simulink model "MPC4"  (R2020b)
settings: Solver=FixedStepAuto  StartTime=0.0  StopTime=10.0  FixedStep=0.01  RelTol=1e-3  EnableMultiTasking=on
model workspace (MAT data in the model file):
  v0_ego = 1
libraries: autolibshared x1, simulink x1
settings Model: Creator=vicgd  LastModifiedBy=vicgd

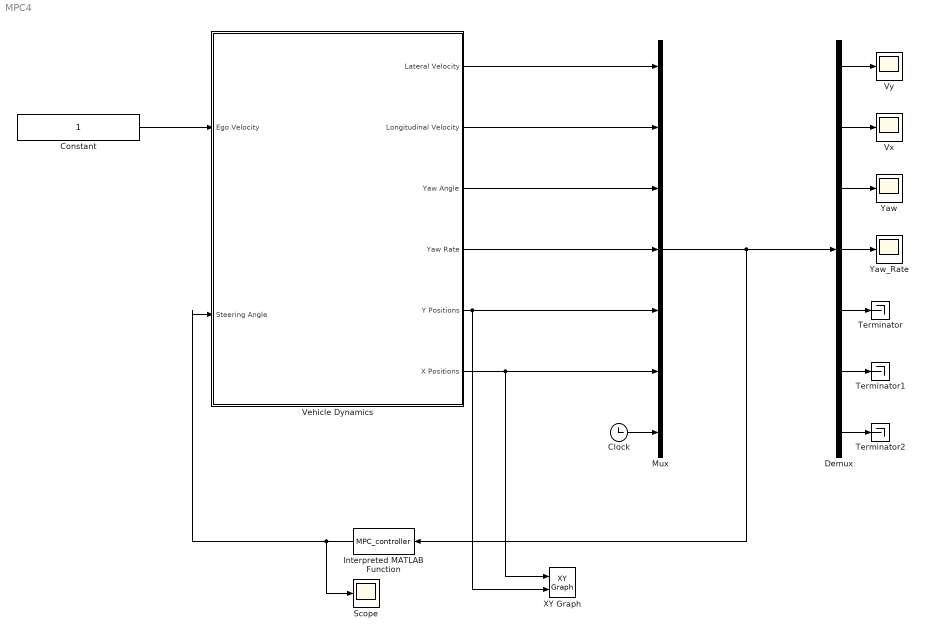
== system MPC4 ==
  Clock : Clock
  Constant : Constant
  Demux : Demux  Outputs=7
  Interpreted MATLAB Function : MATLABFcn  MATLABFcn=MPC_controller  OutputDimensions=1  Output1D=off
  Mux : Mux  Inputs=7
  Scope : Scope
  Terminator : Terminator
  Terminator1 : Terminator
  Terminator2 : Terminator
  Vehicle Dynamics : Subsystem
  Vx : Scope
  Vy : Scope
  XY Graph : simulink/Sinks/XY Graph  xmin=0  xmax=100  ymin=0  ymax=6  st=-1
  Yaw : Scope
  Yaw_Rate : Scope
  wires:
  Mux/1 -> Interpreted MATLAB Function/1, Demux/1
  Clock/1 -> Mux/7
  Vehicle Dynamics/2(Longitudinal Velocity) -> Mux/2
  Vehicle Dynamics/1(Lateral Velocity) -> Mux/1
  Vehicle Dynamics/3(Yaw Angle) -> Mux/3
  Vehicle Dynamics/4(Yaw Rate) -> Mux/4
  Vehicle Dynamics/5(Y Positions) -> XY Graph/2, Mux/5
  Vehicle Dynamics/6(X Positions) -> XY Graph/1, Mux/6
  Demux/1 -> Vy/1
  Demux/2 -> Vx/1
  Demux/3 -> Yaw/1
  Demux/4 -> Yaw_Rate/1
  Interpreted MATLAB Function/1 -> Scope/1, Vehicle Dynamics/2(Steering Angle)
  Constant/1 -> Vehicle Dynamics/1(Ego Velocity)
  Demux/6 -> Terminator1/1
  Demux/7 -> Terminator2/1
  Demux/5 -> Terminator/1

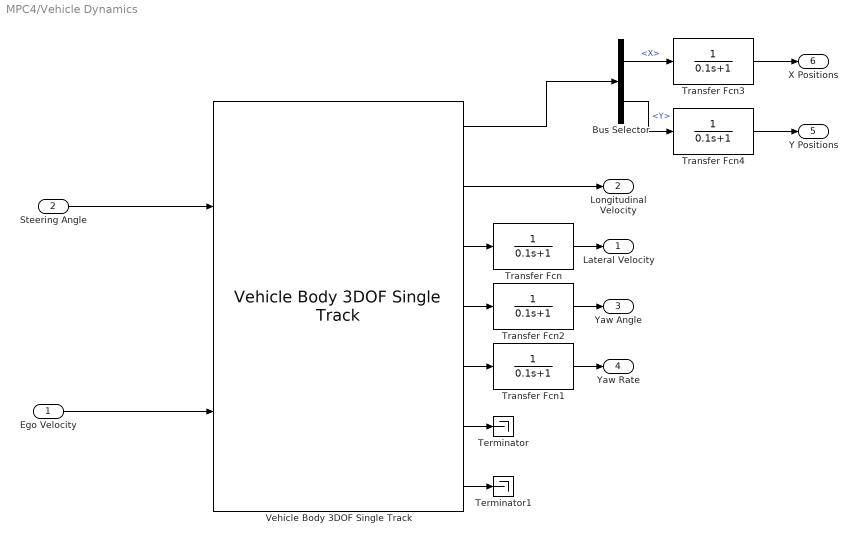
== system MPC4/Vehicle Dynamics ==
  Ego Velocity : Inport
  Steering Angle : Inport  Port=2
  Bus Selector : BusSelector  OutputSignals=InertFrm.Geom.Disp.X,InertFrm.Geom.Disp.Y
  Terminator : Terminator
  Terminator1 : Terminator
  Transfer Fcn{,1..4} (5 alike) : TransferFcn  Denominator=[0.1 1]
  Vehicle Body 3DOF Single Track : autolibshared/Vehicle Body 3DOF Single Track  trackMode=Single (bicycle)  inputMode=External longitudinal velocity  frontSteerMode=on  rearSteerMode=off  windMode=off  muMode=off  extFMode=off  extMMode=off  htchFMode=off  htchMMode=off  extXo=off  extpsio=off  extxdoto=off  extro=off  extYo=off  extTamb=off  extydoto=off  aMode=2  NF=2  NR=2  m=1270  a=1.015  b=1.895  h=0.35  dh=1  hh=0.2  X_o=0  xdot_o=0  CalphaMode=off  sigmaMode=off  d=0  hl=0  w=[1.4,1.4]  Cy_f=1.4e5  Cy_r=8.6e4  sigma_f=.1  sigma_r=.1  alpha_f_brk=[-.1 .1]  Cy_f_data=[-9e3 9e3]  alpha_r_brk=[-.1 .1]  Cy_r_data=[-9e3 9e3]  Y_o=0  ydot_o=0  Izz=1537  psi_o=0  r_o=0  Af=2  Cd=.3  Cl=.1  Cpm=.1  beta_w=[0:0.01:0.3]  Cs=[0:0.03:0.9]  Cym=[0:0.01:0.3]  Pabs=101325  Tair=273  g=9.81  mu=1  xdot_tol=.01  Fznom=5000  Fxtire_sat=7e4  Fytire_sat=7e4  longOff=0  latOff=0  vertOff=0  wrapAng=off
      settings: SourceProductBaseCode=PW,MT,UV,VE,VP
  Lateral Velocity : Outport
  Longitudinal Velocity : Outport  Port=2
  Yaw Angle : Outport  Port=3
  Yaw Rate : Outport  Port=4
  Y Positions : Outport  Port=5
  X Positions : Outport  Port=6
  wires:
  Vehicle Body 3DOF Single Track/3 -> Transfer Fcn/1
  Vehicle Body 3DOF Single Track/4 -> Transfer Fcn2/1
  Vehicle Body 3DOF Single Track/5 -> Transfer Fcn1/1
  Vehicle Body 3DOF Single Track/6 -> Terminator/1
  Vehicle Body 3DOF Single Track/7 -> Terminator1/1
  Ego Velocity/1 -> Vehicle Body 3DOF Single Track/2
  Steering Angle/1 -> Vehicle Body 3DOF Single Track/1
  Vehicle Body 3DOF Single Track/1 -> Bus Selector/1
  Transfer Fcn/1 -> Lateral Velocity/1
  Transfer Fcn2/1 -> Yaw Angle/1
  Transfer Fcn1/1 -> Yaw Rate/1
  Vehicle Body 3DOF Single Track/2 -> Longitudinal Velocity/1
  Transfer Fcn4/1 -> Y Positions/1
  Transfer Fcn3/1 -> X Positions/1
  Bus Selector/2 -> Transfer Fcn4/1  "<Y>"
  Bus Selector/1 -> Transfer Fcn3/1  "<X>"
